simulink model "lab02"  (R2025a)
settings: Solver=VariableStepAuto  StartTime=0.0  StopTime=300  RelTol=1e-4
settings Model: Creator=razrab-ytka  LastModifiedBy=grigorijtomczuk
settings SolverCC: AlgebraicLoopSolver=TrustRegion
settings DebuggingCC: ArithmeticOperatorsInVariantConditions=warning
settings SFSimCC: CustomCodeUndefinedFunction=UseInterfaceOnly
settings RTWCC: GPUComputeCapability=3.5
settings CodeAppCC: StateflowObjectComments=on

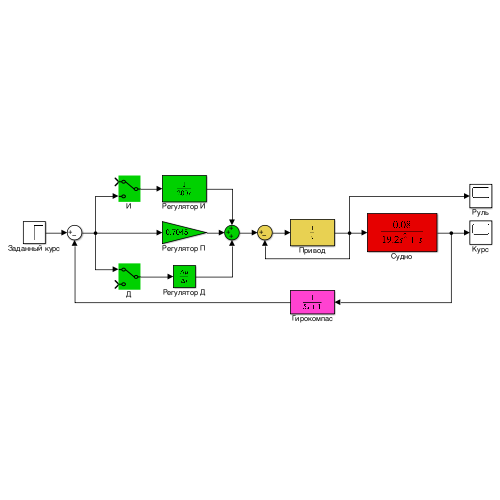
[thumbnail: Simulink's stored preview of the top-level diagram]
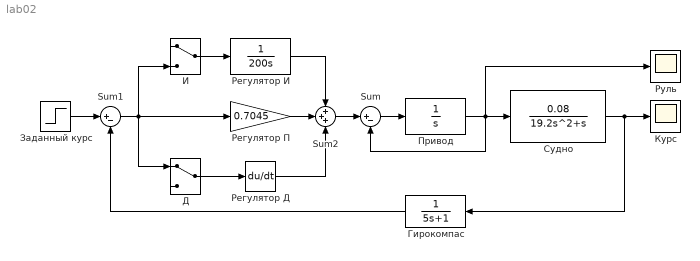
== system lab02 ==
  Sum : Sum  Inputs=|+-
  Sum1 : Sum  Inputs=|+-
  Sum2 : Sum  Inputs=+++
  Гирокомпас : TransferFcn  Denominator=[5 1]
  Д : ManualSwitch
  Заданный курс : Step  Time=0  After=10  SampleTime=0
  И : ManualSwitch
  Курс : Scope
      settings: ActiveDisplayYMinimum=-1.6333131175709545  ActiveDisplayYMaximum=14.699818058138595
  Привод : TransferFcn  Denominator=[1 0]
  Регулятор Д : Derivative
  Регулятор И : TransferFcn  Denominator=[200 0]
  Регулятор П : Gain  Gain=0.7045
  Руль : Scope
      settings: ActiveDisplayYMinimum=-3.575451477071605  ActiveDisplayYMaximum=8.1533933111761741
  Судно : TransferFcn  Numerator=[0.08]  Denominator=[19.2 1 0]
  wires:
  Sum/1 -> Привод/1
  Судно/1 -> Гирокомпас/1, Курс/1
  Гирокомпас/1 -> Sum1/2
  Регулятор И/1 -> Sum2/1
  Sum2/1 -> Sum/1
  Sum1/1 -> И/2, Д/1, Регулятор П/1
  Заданный курс/1 -> Sum1/1
  И/1 -> Регулятор И/1
  Привод/1 -> Судно/1, Руль/1, Sum/2
  Регулятор Д/1 -> Sum2/3
  Регулятор П/1 -> Sum2/2
  Д/1 -> Регулятор Д/1
